simulink model "graphical_function"  (Simulink 7.6)
settings: Solver=FixedStepDiscrete  StartTime=0.0  StopTime=10.0  FixedStep=1  RelTol=1e-3
settings Model: Creator=ksmyth  LastModifiedBy=c2wt
settings OptimizationCC: InitFltsAndDblsToZero=on
settings DebuggingCC: SaveWithParameterizedLinksMsg=none  StrictBusMsg=Warning
settings SFSimCC: SimParseCustomCode=off
settings GRTTargetCC: TargetFcnLib=ansi_tfl_tmw.mat

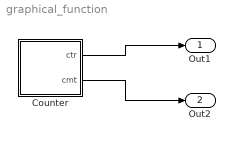
== system graphical_function ==
  Counter : Stateflow chart  TreatAsAtomicUnit=on
  Out1 : Outport
  Out2 : Outport  Port=2
  wires:
  Counter/1(ctr) -> Out1/1
  Counter/2(cmt) -> Out2/1

== stateflow chart Counter ==
  state s1
  state y = mod2(x) [function]
    (default) -> (junction 5)
    (junction 5) -> (junction 6) [order 1] : [int32(x/2)*2 == x]{y = 1;}
    (junction 5) -> (junction 7) [order 2] : {y = 0;}
  (default) -> s1
  (junction 11) -> s1 [order 1] : [ctr < 4] / ctr = ctr+1;
  (junction 11) -> s1 [order 2] : / ctr = -2; cmt = -1;
  s1 -> (junction 8)
  (junction 8) -> (junction 9) : { temp = mod2( ctr ); }
  (junction 9) -> (junction 10) [order 1] : [temp == 1]{cmt = cmt + 1;}
  (junction 9) -> (junction 11) [order 2]
  (junction 10) -> (junction 11)
  data: x function_input int32; y function_output double; ctr output double =1; cmt output double; temp local double
